simulink model "revisedLaneChange"  (R2018b)
settings: Solver=FixedStepAuto  StartTime=0.0  StopTime=40  FixedStep=0.01  RelTol=1e-3
libraries: simulink x1
settings Model: Creator=jasprit  LastModifiedBy=jasprit

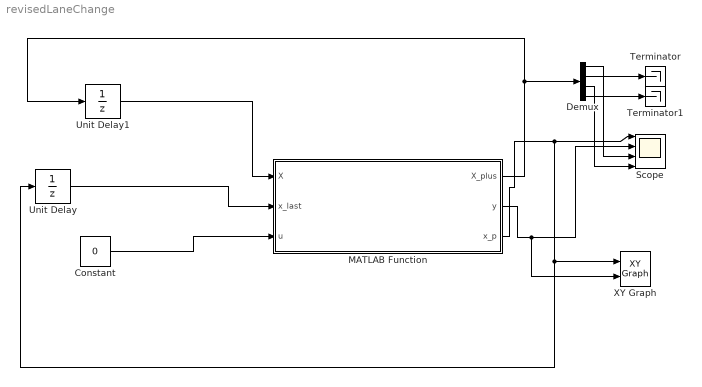
== system revisedLaneChange ==
  Constant : Constant  Value=0  SampleTime=-1
  Demux : Demux
  MATLAB Function : MATLAB Function  TreatAsAtomicUnit=on
  Scope : Scope  NumInputPorts=4
  Terminator : Terminator
  Terminator1 : Terminator
  Unit Delay : UnitDelay  SampleTime=-1
  Unit Delay1 : UnitDelay  InitialCondition=[0;10;0;0]  SampleTime=-1
  XY Graph : simulink/Sinks/XY Graph  xmin=-1  xmax=200  ymin=-5  ymax=5  st=-1
  wires:
  Unit Delay/1 -> MATLAB Function/2(x_last)
  MATLAB Function/3(x_p) -> Unit Delay/1, XY Graph/1, Scope/1
  Constant/1 -> MATLAB Function/3(u)
  MATLAB Function/2(y) -> XY Graph/2, Scope/2
  Unit Delay1/1 -> MATLAB Function/1(X)
  MATLAB Function/1(X_plus) -> Demux/1, Unit Delay1/1
  Demux/2 -> Terminator/1
  Demux/4 -> Terminator1/1
  Demux/1 -> Scope/3
  Demux/3 -> Scope/4

== matlab function revisedLaneChange/MATLAB Function ==
  data: X_plus output; X input; x_last input; u input; y output; x_p output
function [X_plus,y, x_p] = sinusoidalLeftLaneChangeRevised(X, x_last, u)
    Ts = 0.01;
    v = 10;
    x_p = x_last + X(2) * Ts;
    L = 100;    
    w = pi/L;
    A = 3.5/2;
    y = -A * cos(w*x_p) + A + u;
    
    f31 = A*w*w*X(2)*X(2)*cos(w*X(1));
    f32 = A*w*sin(w*X(1));
    f41 = -A*(w*v)^3*sin(w*X(1));
    f42 = 2*A*w*w*v*cos(w*X(1));
    F = [0 1 0 0; ...
        0 0 0 0; ...
        f31 f32 0 0; ...
        0 2*A*w*w*X(2) -w*w*X(2)^2 0];
%         f41 f42 0 0]; 
    
%     Bd = [0; 0; A; 0];
    Bd = [0; 0; 0; 0];
    Fd = expm(F*Ts);
    X_plus = Fd*X + Bd*Ts;
end
